simulink model "State_obs"  (R2020b)
settings: Solver=VariableStepAuto  StartTime=0.0  StopTime=10.0  RelTol=1e-3
values from neighbouring files (symbols this model uses):
  Ts = 1e-2    (= 0.01)    [balrob_params.m]
undefined symbols (not defined in the file or in its folder): C_gain, denHw, denLPFz, DiscIntNeverNeededParam, gbox, numHw, numLPFz, sens, T
settings Model: Creator=Andrea  LastModifiedBy=Andrea
settings DebuggingCC: SFMachineParentedDataDiag=error

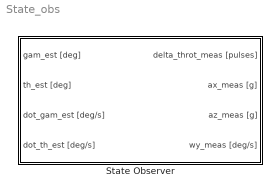
== system State_obs ==
  State Observer : Subsystem

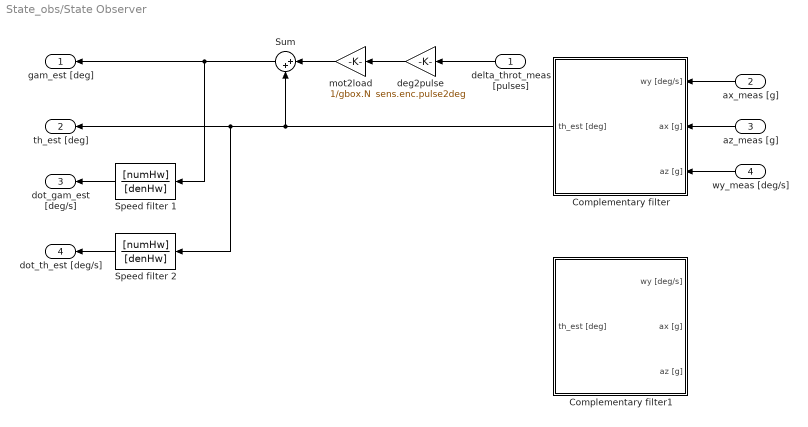
== system State_obs/State Observer ==
  "delta_throt_meas [pulses] " : Inport
  "ax_meas [g] " : Inport  Port=2
  "az_meas [g] " : Inport  Port=3
  wy_meas [deg/s] : Inport  Port=4
  Complementary filter : Subsystem
  Complementary filter1 : Subsystem
  Speed filter 1 : DiscreteTransferFcn  Numerator=[numHw]  Denominator=[denHw]
  Speed filter 2 : DiscreteTransferFcn  Numerator=[numHw]  Denominator=[denHw]
  Sum : Sum  Inputs=|++
  deg2pulse : Gain  Gain=sens.enc.pulse2deg
  mot2load : Gain  Gain=1/gbox.N
  gam_est [deg] : Outport
  th_est [deg] : Outport  Port=2
  dot_gam_est [deg/s] : Outport  Port=3
  dot_th_est [deg/s] : Outport  Port=4
  wires:
  "ax_meas [g] "/1 -> Complementary filter/1(wy [deg/s])
  "az_meas [g] "/1 -> Complementary filter/2("ax [g] ")
  wy_meas [deg/s]/1 -> Complementary filter/3("az [g] ")
  deg2pulse/1 -> mot2load/1
  "delta_throt_meas [pulses] "/1 -> deg2pulse/1
  mot2load/1 -> Sum/1
  Complementary filter/1("th_est [deg] ") -> Sum/2, Speed filter 2/1, th_est [deg]/1
  Sum/1 -> Speed filter 1/1, gam_est [deg]/1
  Speed filter 1/1 -> dot_gam_est [deg/s]/1
  Speed filter 2/1 -> dot_th_est [deg/s]/1

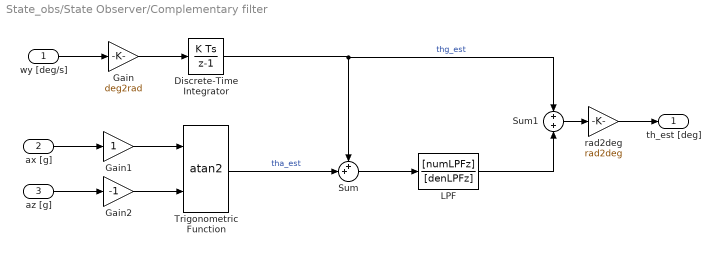
== system State_obs/State Observer/Complementary filter ==
  wy [deg/s] : Inport
  "ax [g] " : Inport  Port=2
  "az [g] " : Inport  Port=3
  Discrete-Time Integrator : DiscreteIntegrator  gainval=1  SampleTime=Ts  ICPrevOutput=DiscIntNeverNeededParam  ICPrevScaledInput=DiscIntNeverNeededParam
  Gain : Gain  Gain=deg2rad
  Gain1 : Gain
  Gain2 : Gain  Gain=-1
  LPF : DiscreteTransferFcn  Numerator=[numLPFz]  Denominator=[denLPFz]
  Sum : Sum  Inputs=++|
  Sum1 : Sum
  Trigonometric Function : Trigonometry  Operator=atan2
  rad2deg : Gain  Gain=rad2deg
  "th_est [deg] " : Outport
  wires:
  "az [g] "/1 -> Gain2/1
  "ax [g] "/1 -> Gain1/1
  wy [deg/s]/1 -> Gain/1
  Gain/1 -> Discrete-Time Integrator/1
  Gain2/1 -> Trigonometric Function/2
  Gain1/1 -> Trigonometric Function/1
  Trigonometric Function/1 -> Sum/2  "tha_est"
  Discrete-Time Integrator/1 -> Sum1/1, Sum/1  "thg_est"
  rad2deg/1 -> "th_est [deg] "/1
  Sum1/1 -> rad2deg/1
  Sum/1 -> LPF/1
  LPF/1 -> Sum1/2

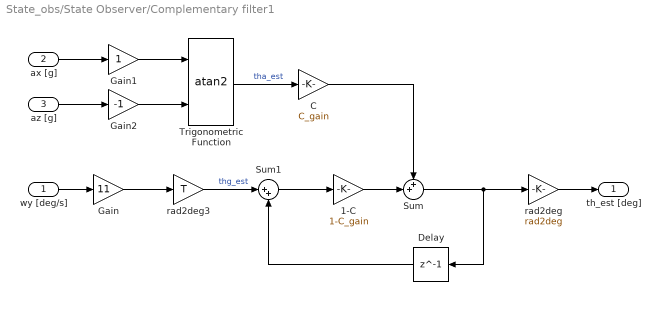
== system State_obs/State Observer/Complementary filter1 ==
  wy [deg/s] : Inport
  "ax [g] " : Inport  Port=2
  "az [g] " : Inport  Port=3
  1-C : Gain  Gain=1-C_gain
  C : Gain  Gain=C_gain
  Delay : Delay  DelayLength=1
  Gain : Gain  Gain=11
  Gain1 : Gain
  Gain2 : Gain  Gain=-1
  Sum : Sum  Inputs=++|
  Sum1 : Sum  Inputs=|++
  Trigonometric Function : Trigonometry  Operator=atan2
  rad2deg : Gain  Gain=rad2deg
  rad2deg3 : Gain  Gain=T
  "th_est [deg] " : Outport
  wires:
  "az [g] "/1 -> Gain2/1
  "ax [g] "/1 -> Gain1/1
  wy [deg/s]/1 -> Gain/1
  Gain/1 -> rad2deg3/1
  Gain2/1 -> Trigonometric Function/2
  Gain1/1 -> Trigonometric Function/1
  rad2deg/1 -> "th_est [deg] "/1
  Trigonometric Function/1 -> C/1  "tha_est"
  C/1 -> Sum/1
  1-C/1 -> Sum/2
  Sum/1 -> Delay/1, rad2deg/1
  Delay/1 -> Sum1/2
  rad2deg3/1 -> Sum1/1  "thg_est"
  Sum1/1 -> 1-C/1
